simulink model "down"  (R2018b)
settings: Solver=VariableStepAuto  StartTime=0.0  StopTime=20  RelTol=1e-3
libraries: commrandsrc3 x1
settings Model: Creator=user  LastModifiedBy=user

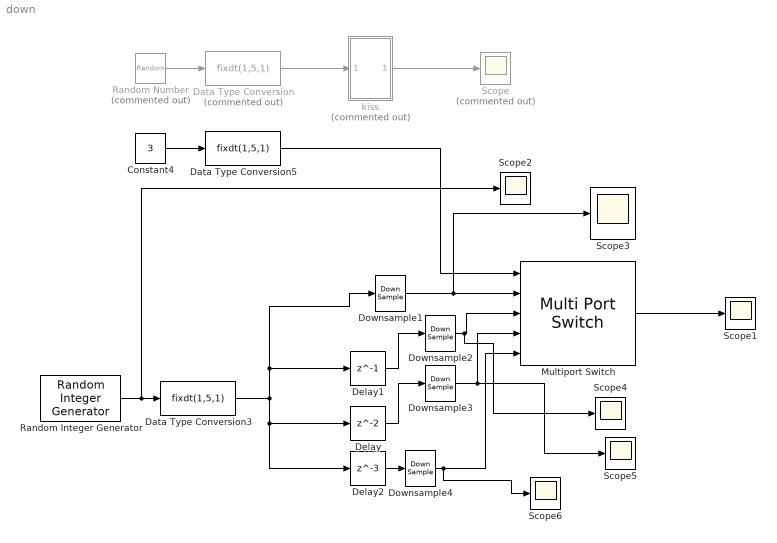
== system down ==
  Constant4 : Constant  Value=3
  Data Type Conversion : DataTypeConversion  Commented=on  OutDataTypeStr=fixdt(1,5,1)  RndMeth=Round  SaturateOnIntegerOverflow=on
  Data Type Conversion3 : DataTypeConversion  OutDataTypeStr=fixdt(1,5,1)  RndMeth=Round  SaturateOnIntegerOverflow=on
  Data Type Conversion5 : DataTypeConversion  OutDataTypeStr=fixdt(1,5,1)  RndMeth=Round  SaturateOnIntegerOverflow=on
  Delay : Delay
  Delay1 : Delay  DelayLength=1
  Delay2 : Delay  DelayLength=3
  Downsample{1..4} (4 alike) : DownSample  N=4  RateOptions=Allow multirate processing
  Multiport Switch : MultiPortSwitch  Inputs=4
  Random Number : RandomNumber  Commented=on  SampleTime=0.1
  Random Integer Generator : commrandsrc3/Random Integer Generator  SetSize=4  SeedSource=Auto  Seed=0  SampleTime=1  SamplesPerFrame=1  OutputDataType=double  SimulateUsing=Interpreted execution
  Scope : Scope  Commented=on
  Scope{1..6} (6 alike) : Scope
  "kiss " : Subsystem  Commented=on
  wires:
  Random Number/1 -> Data Type Conversion/1
  Data Type Conversion/1 -> "kiss "/1(In1)
  "kiss "/1(Out1) -> Scope/1
  Constant4/1 -> Data Type Conversion5/1
  Data Type Conversion3/1 -> Delay1/1, Downsample1/1, Delay2/1, Delay/1
  Multiport Switch/1 -> Scope1/1
  Delay2/1 -> Downsample4/1
  Delay/1 -> Downsample3/1
  Delay1/1 -> Downsample2/1
  Downsample1/1 -> Scope3/1, Multiport Switch/2
  Downsample2/1 -> Scope4/1, Multiport Switch/3
  Downsample3/1 -> Scope5/1, Multiport Switch/4
  Downsample4/1 -> Multiport Switch/5, Scope6/1
  Data Type Conversion5/1 -> Multiport Switch/1
  Random Integer Generator/1 -> Scope2/1, Data Type Conversion3/1

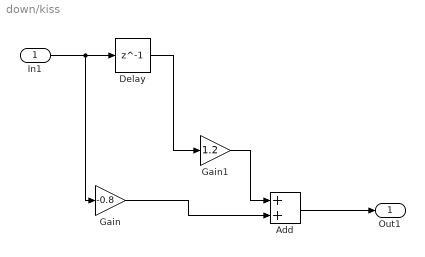
== system down/kiss  ==
  In1 : Inport
  Add : Sum
  Delay : Delay  DelayLength=1
  Gain : Gain  Gain=-0.8
  Gain1 : Gain  Gain=1.2
  Out1 : Outport
  wires:
  In1/1 -> Gain/1, Delay/1
  Delay/1 -> Gain1/1
  Gain1/1 -> Add/1
  Gain/1 -> Add/2
  Add/1 -> Out1/1
